simulink model "WTTSRTracker_UncertaintyStability"  (R2021a)
settings: Solver=VariableStepDiscrete  StartTime=0.0  StopTime=TMax  MaxStep=Ts  RelTol=1e-3
values from neighbouring files (symbols this model uses):
  CpUncertaintyFactor = 1    [WTTSRTracker_UncertaintyStability_init.m]
  T = loadturbineconstants('NREL5MW')    [WTTSRTracker_UncertaintyStability_init.m]
  Tg0 = 2.4e4    (= 24000)    [WTTSRTracker_UncertaintyStability_init.m]
  Ts = 0.01    [WTTSRTracker_UncertaintyStability_init.m]
  TSR_Ki = -50    [WTTSRTracker_UncertaintyStability_init.m]
  TSR_Kp = -0    (= 0)    [WTTSRTracker_UncertaintyStability_init.m]
  V0 = 9    [WTTSRTracker_UncertaintyStability_init.m]
  WSE_Ki = 1    [WTTSRTracker_UncertaintyStability_init.m]
  WSE_Kp = 10    [WTTSRTracker_UncertaintyStability_init.m]
undefined symbols (not defined in the file or in its folder): rads2rpm
libraries: DRC_SimulinkLibrary x5
settings Model: PacingRate=79  Creator=Sebastiaan  LastModifiedBy=sebastiaanmuld

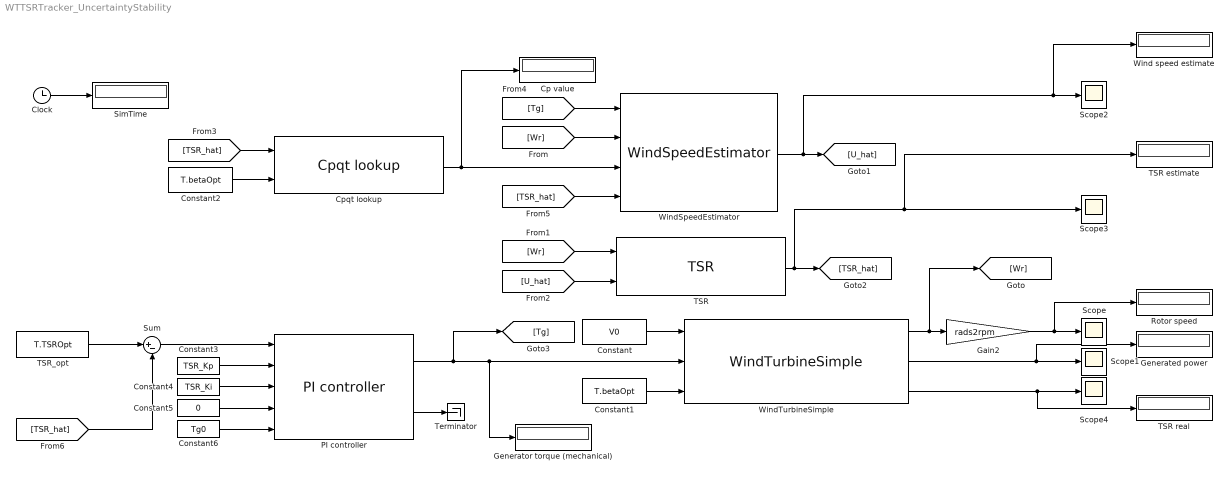
== system WTTSRTracker_UncertaintyStability ==
  Clock : Clock
  Constant : Constant  Value=V0
  Constant1 : Constant  Value=T.betaOpt
  Constant2 : Constant  Value=T.betaOpt
  Constant3 : Constant  Value=TSR_Kp
  Constant4 : Constant  Value=TSR_Ki
  Constant5 : Constant  Value=0
  Constant6 : Constant  Value=Tg0
  Cp value : Display
  Cpqt lookup : DRC_SimulinkLibrary/Cpqt lookup  CpqtGrid=T.Cp*CpUncertaintyFactor  TSRVector=T.CTSR  PitchVector=T.CPitch
  Gain2 : Gain  Gain=rads2rpm
  Generated power : Display
  Generator torque (mechanical) : Display
  PI controller : DRC_SimulinkLibrary/PI controller  minSatValue=T.Tg_min  maxSatValue=T.Tg_max  Ts=Ts
  Rotor speed : Display
  Scope{,1..4} (5 alike) : Scope
  SimTime : Display
  Sum : Sum  Inputs=|+-
  TSR : DRC_SimulinkLibrary/TSR  RotorRadius=T.R
  TSR estimate : Display
  TSR real : Display
  TSR_opt : Constant  Value=T.TSROpt
  Terminator : Terminator
  Wind speed estimate : Display
  WindSpeedEstimator : DRC_SimulinkLibrary/WindSpeedEstimator  R=T.R  TrMax=T.Tg_max*T.G  G=T.G  JLss=T.Jlss  rho=T.rho  Kp=WSE_Kp  Ki=WSE_Ki  omega_r_0=Wr0  V0=V0  Ts=Ts
  WindTurbineSimple : DRC_SimulinkLibrary/WindTurbineSimple  R=T.R  rho=T.rho  TMax=T.Tg_max*T.G  JWr=T.Jlss  G=T.G  Wr0=Wr0  CpArray=T.Cp  TSRVec=T.CTSR  betaVec=T.CPitch
  wires:
  Constant/1 -> WindTurbineSimple/1
  Constant1/1 -> WindTurbineSimple/3
  Gain2/1 -> Rotor speed/1, Scope/1
  WindTurbineSimple/1 -> [Wr], Gain2/1
  WindTurbineSimple/2 -> Generated power/1, Scope1/1
  Clock/1 -> SimTime/1
  [Wr] -> WindSpeedEstimator/2
  PI controller/1 -> Generator torque (mechanical)/1, WindTurbineSimple/2, [Tg]
  Cpqt lookup/1 -> Cp value/1, WindSpeedEstimator/3
  [Wr] -> TSR/1
  WindSpeedEstimator/1 -> Wind speed estimate/1, Scope2/1, [U_hat]
  [U_hat] -> TSR/2
  TSR/1 -> TSR estimate/1, Scope3/1, [TSR_hat]
  [TSR_hat] -> Cpqt lookup/1
  Constant2/1 -> Cpqt lookup/2
  [Tg] -> WindSpeedEstimator/1
  [TSR_hat] -> WindSpeedEstimator/4
  TSR_opt/1 -> Sum/1
  Sum/1 -> PI controller/1
  PI controller/2 -> Terminator/1
  Constant3/1 -> PI controller/2
  Constant4/1 -> PI controller/3
  Constant5/1 -> PI controller/4
  Constant6/1 -> PI controller/5
  [TSR_hat] -> Sum/2
  WindTurbineSimple/3 -> TSR real/1, Scope4/1
